simulink model "F16BlockSYM"  (R2012b)
settings: Solver=ode5  StartTime=0.0  StopTime=TFinal  FixedStep=delta_T  RelTol=1e-3
values from neighbouring files (symbols this model uses):
  DisAil_1 = AileronDis    (= 0)    [runF16Sim.m]
  DisAil_2 = -2*AileronDis    (= 0)    [runF16Sim.m]
  DisAil_3 = AileronDis    (= 0)    [runF16Sim.m]
  DisEle_1 = ElevatorDis    (= 0)    [runF16Sim.m]
  DisEle_2 = -2*ElevatorDis    (= 0)    [runF16Sim.m]
  DisEle_3 = ElevatorDis    (= 0)    [runF16Sim.m]
  DisRud_1 = RudderDis    (= 0)    [runF16Sim.m]
  DisRud_2 = -2*RudderDis    (= 0)    [runF16Sim.m]
  DisRud_3 = RudderDis    (= 0)    [runF16Sim.m]
  fi_flag_Simulink = 1    [runF16Sim.m]
  trim_control = [UX(2);UX(5);UX(6)]    [trim_F16_fast.m]
  trim_state = xu(1:13)    [trim_F16_fast.m]
  trim_throttle = UX(1)    [trim_F16_fast.m]
libraries: F16_Actuator_Library x4, aerolibtransform2 x1, aerolibatmos2 x1
settings Model: ExtModeAutoUpdateStatusClock=off  Creator=keviczky  LastModifiedBy=David
settings DataIOCC: Decimation=50  LimitDataPoints=off  SignalLoggingSaveFormat=ModelDataLogs  SignalLoggingName=sigsOut
settings OptimizationCC: BooleanDataType=off  InlineInvariantSignals=on
settings DebuggingCC: SaveWithParameterizedLinksMsg=none  SignalResolutionControl=TryResolveAllWithWarning  SolverPrmCheckMsg=none  MultiTaskDSMMsg=warning  MultiTaskCondExecSysMsg=none  StrictBusMsg=None
settings HardwareCC: TargetUnknown=on
settings RTWCC: IncludeERTFirstTime=on
settings GRTTargetCC: CombineOutputUpdateFcns=off  GRTInterface=on

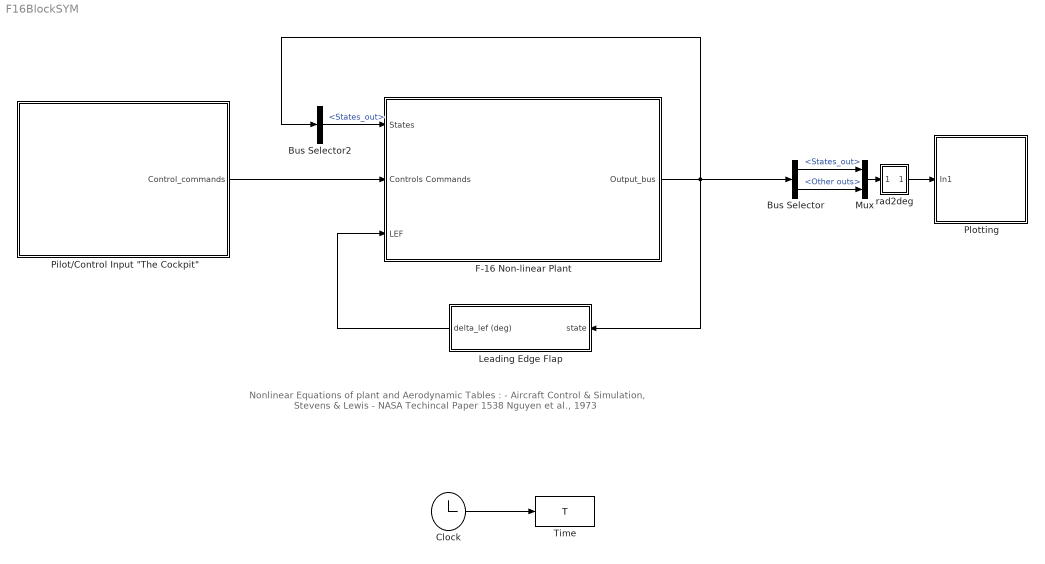
== system F16BlockSYM ==
  note: Nonlinear Equations of plant and Aerodynamic Tables :
      | - Aircraft Control & Simulation, Stevens & Lewis
      | - NASA Techincal Paper 1538 Nguyen et al., 1973
  Bus Selector : BusSelector  OutputSignals=States_out,Other outs
  Bus Selector2 : BusSelector  OutputSignals=States_out
  Clock : Clock
      settings: Decimation=50
  F-16 Non-linear Plant : Subsystem
      mask Display:
      | image(imread('f16.jpg'))
      | port_label('output', 1, 'Out_bus')
      | port_label('input', 1, 'State_feedback')
      | port_label('input', 2, 'Control_Commands')
      | port_label('input', 3, 'LEF_def')
  Leading Edge Flap : Subsystem
  Mux : Mux  Inputs=2
  "Pilot/Control Input \"The Cockpit\"" : Subsystem
      mask Display:
      | image(imread('F-16-Cockpit.jpg'))
      | port_label('output', 1, 'Control_commands')
  Plotting : Subsystem
      mask Display: image(imread('f16output.jpg'))
  Time : ToWorkspace  VariableName=T  SampleTime=-1
      settings: Decimation=100
  rad2deg : Subsystem
  wires:
  "Pilot/Control Input \"The Cockpit\""/1(Control_commands) -> F-16 Non-linear Plant/2(Controls Commands)
  Clock/1 -> Time/1
  rad2deg/1(Out1) -> Plotting/1(In1)
  Bus Selector/1 -> Mux/1  "<States_out>"
  Bus Selector/2 -> Mux/2  "<Other outs>"
  Mux/1 -> rad2deg/1(In1)
  F-16 Non-linear Plant/1(Output_bus) -> Leading Edge Flap/1(state), Bus Selector2/1, Bus Selector/1
  Bus Selector2/1 -> F-16 Non-linear Plant/1(States)  "<States_out>"
  Leading Edge Flap/1(delta_lef (deg)) -> F-16 Non-linear Plant/3(LEF)

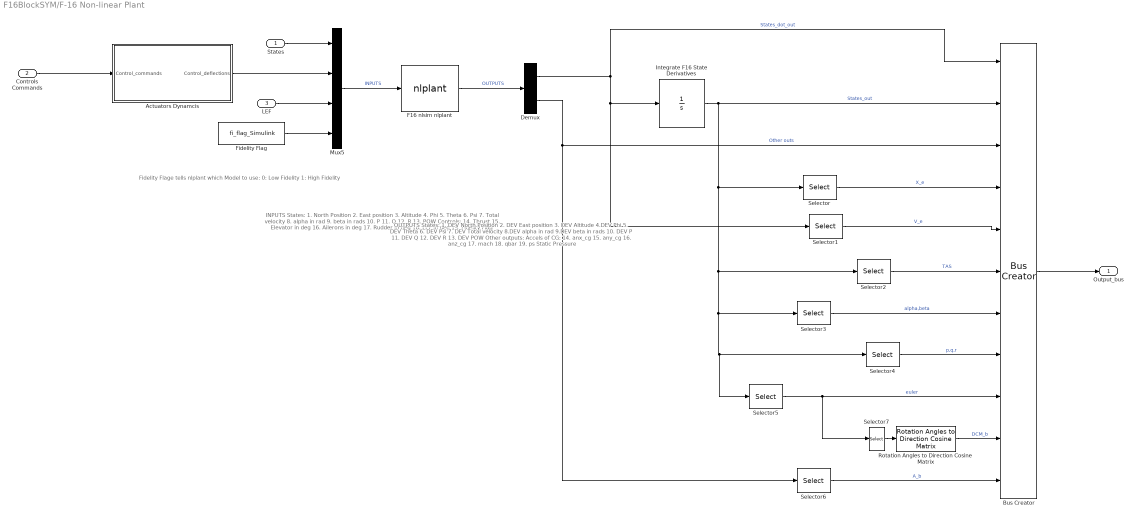
== system F16BlockSYM/F-16 Non-linear Plant ==
  note: INPUTS
      | States:
      | 1. North Position
      | 2. East position
      | 3. Altitude
      | 4. Phi
      | 5. Theta
      | 6. Psi
      | 7. Total velocity
      | 8. alpha in rad
      | 9. beta in rads
      | 10. P
      | 11. Q
      | 12. R
      | 13. POW
      |
      | Controls:
      | 14. Thrust
      | 15. Elevator in deg
      | 16. Ailerons in deg
      | 17. Rudder in deg
      | 18. LEF in deg
      |
      | 19. Fidelity Flag
  note: OUTPUTS
      | States:
      | 1. DEV North Position
      | 2. DEV East position
      | 3. DEV Altitude
      | 4.DEV  Phi
      | 5. DEV Theta
      | 6. DEV Psi
      | 7. DEV Total velocity
      | 8.DEV alpha in rad
      | 9.DEV  beta in rads
      | 10. DEV P
      | 11. DEV Q
      | 12. DEV R
      | 13. DEV POW
      |
      | Other outputs:
      | Accels of CG:
      | 14. anx_cg
      | 15. any_cg
      | 16. anz_cg
      | 17. mach
      | 18. qbar
      | 19. ps   Static Pressure
  note: Fidelity Flage tells nlplant
      | which Model to use:
      | 0: Low Fidelity
      | 1: High Fidelity
  States : Inport
  Controls Commands : Inport  Port=2
  LEF : Inport  Port=3
  Actuators Dynamcis : Subsystem  TreatAsAtomicUnit=on
  Bus Creator : BusCreator  Inputs=11
  Demux : Demux  Outputs=[13 6]
  F16 nlsim nlplant : MATLABFcn  MATLABFcn=nlplant  OutputDimensions=19  OutputSignalType=real
  Fidelity Flag : Constant  Value=fi_flag_Simulink
  Integrate F16 State Derivatives : Integrator  InitialCondition=trim_state
  Mux5 : Mux  Inputs=[13 4 1 1]
  Rotation Angles to Direction Cosine Matrix : aerolibtransform2/Rotation Angles to Direction Cosine Matrix  rotationOrder=ZYX
  Selector : Selector  InputPortWidth=13  IndexOptions=Index vector (dialog)  Indices=[1:3]  OutputSizes=1
  Selector1 : Selector  InputPortWidth=13  IndexOptions=Index vector (dialog)  Indices=[1:3]  OutputSizes=1
  Selector2 : Selector  InputPortWidth=13  IndexOptions=Index vector (dialog)  Indices=[7]  OutputSizes=1
  Selector3 : Selector  InputPortWidth=13  IndexOptions=Index vector (dialog)  Indices=[8:9]  OutputSizes=1
  Selector4 : Selector  InputPortWidth=13  IndexOptions=Index vector (dialog)  Indices=[10:12]  OutputSizes=1
  Selector5 : Selector  InputPortWidth=13  IndexOptions=Index vector (dialog)  Indices=[4:6]  OutputSizes=1
  Selector6 : Selector  InputPortWidth=6  IndexOptions=Index vector (dialog)  Indices=[1:3]  OutputSizes=1
  Selector7 : Selector  InputPortWidth=3  IndexOptions=Index vector (dialog)  Indices=[3 2 1]  OutputSizes=1
  Output_bus : Outport
  wires:
  Demux/1 -> Selector1/1, Integrate F16 State Derivatives/1, Bus Creator/1  "States_dot_out"
  Selector/1 -> Bus Creator/4  "X_e"
  Selector1/1 -> Bus Creator/5  "V_e"
  Selector2/1 -> Bus Creator/6  "TAS"
  Selector3/1 -> Bus Creator/7  "alpha,beta"
  Selector4/1 -> Bus Creator/8  "p,q,r"
  Selector5/1 -> Selector7/1, Bus Creator/9  "euler"
  Selector6/1 -> Bus Creator/11  "A_b"
  Demux/2 -> Selector6/1, Bus Creator/3  "Other outs"
  Selector7/1 -> Rotation Angles to Direction Cosine Matrix/1
  Integrate F16 State Derivatives/1 -> Selector5/1, Selector4/1, Selector3/1, Selector2/1, Selector/1, Bus Creator/2  "States_out"
  Rotation Angles to Direction Cosine Matrix/1 -> Bus Creator/10  "DCM_b"
  Bus Creator/1 -> Output_bus/1
  Fidelity Flag/1 -> Mux5/4
  LEF/1 -> Mux5/3
  Controls Commands/1 -> Actuators Dynamcis/1(Control_commands)
  States/1 -> Mux5/1
  Mux5/1 -> F16 nlsim nlplant/1  "INPUTS"
  F16 nlsim nlplant/1 -> Demux/1  "OUTPUTS"
  Actuators Dynamcis/1(Control_deflections) -> Mux5/2

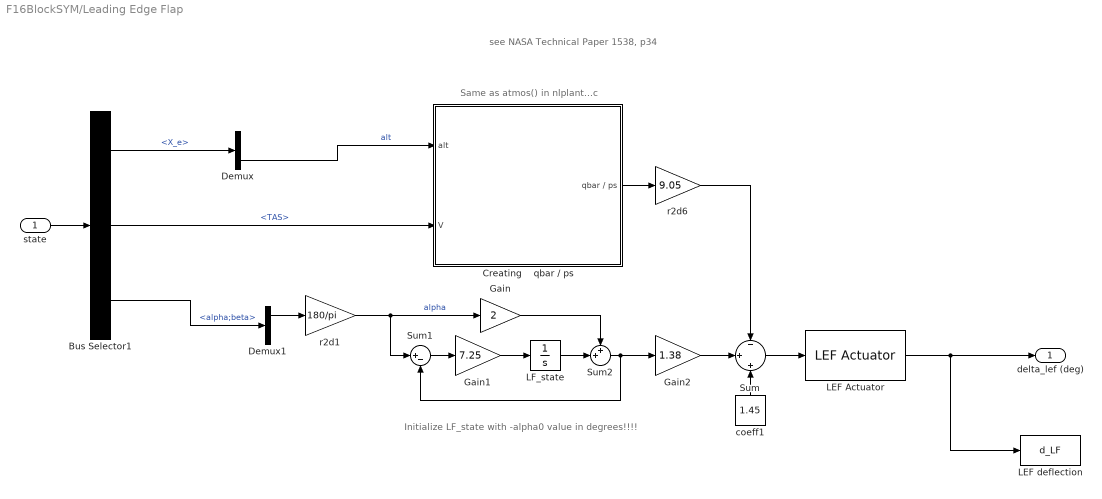
== system F16BlockSYM/Leading Edge Flap ==
  note: see NASA Technical Paper 1538, p34
  note: Same as atmos() in nlplant...c
  note: Initialize LF_state with -alpha0 value in degrees!!!!
  state : Inport
  Bus Selector1 : BusSelector  OutputSignals=X_e,TAS,alpha;beta
  Creating    qbar / ps : Subsystem
  Demux : Demux  Outputs=3
  Demux1 : Demux  Outputs=2
  Gain : Gain  Gain=2  SaturateOnIntegerOverflow=on  OutDataTypeStr=Inherit: Same as input  ParamDataTypeStr=Inherit: Same as input
  Gain1 : Gain  Gain=7.25  SaturateOnIntegerOverflow=on  OutDataTypeStr=Inherit: Same as input  ParamDataTypeStr=Inherit: Same as input
  Gain2 : Gain  Gain=1.38  SaturateOnIntegerOverflow=on  OutDataTypeStr=Inherit: Same as input  ParamDataTypeStr=Inherit: Same as input
  LEF Actuator : F16_Actuator_Library/LEF Actuator
  LEF deflection : ToWorkspace  VariableName=d_LF  SampleTime=-1
      settings: Decimation=100
  LF_state : Integrator  InitialCondition=-trim_state(8)*180/pi
  Sum : Sum  Inputs=-|+|+  SaturateOnIntegerOverflow=on  InputSameDT=on  OutDataTypeStr=Inherit: Same as first input
  Sum1 : Sum  Inputs=|+-  SaturateOnIntegerOverflow=on  InputSameDT=on  OutDataTypeStr=Inherit: Same as first input
  Sum2 : Sum  Inputs=++|  SaturateOnIntegerOverflow=on  InputSameDT=on  OutDataTypeStr=Inherit: Same as first input
  coeff1 : Constant  Value=1.45
  r2d1 : Gain  Gain=180/pi  SaturateOnIntegerOverflow=on  OutDataTypeStr=Inherit: Same as input  ParamDataTypeStr=Inherit: Same as input
  r2d6 : Gain  Gain=9.05  SaturateOnIntegerOverflow=on  OutDataTypeStr=Inherit: Same as input  ParamDataTypeStr=Inherit: Same as input
  delta_lef (deg) : Outport
  wires:
  LEF Actuator/1 -> LEF deflection/1, delta_lef (deg)/1
  Sum/1 -> LEF Actuator/1
  state/1 -> Bus Selector1/1
  Sum1/1 -> Gain1/1
  Gain1/1 -> LF_state/1
  Gain/1 -> Sum2/1
  Gain2/1 -> Sum/2
  Demux1/1 -> r2d1/1
  coeff1/1 -> Sum/3
  Sum2/1 -> Sum1/2, Gain2/1
  LF_state/1 -> Sum2/2
  r2d1/1 -> Sum1/1, Gain/1  "alpha"
  Bus Selector1/2 -> Creating    qbar / ps/2(V)  "<TAS>"
  Creating    qbar / ps/1(qbar / ps) -> r2d6/1
  r2d6/1 -> Sum/1
  Demux/3 -> Creating    qbar / ps/1(alt)  "alt"
  Bus Selector1/1 -> Demux/1  "<X_e>"
  Bus Selector1/3 -> Demux1/1  "<alpha;beta>"

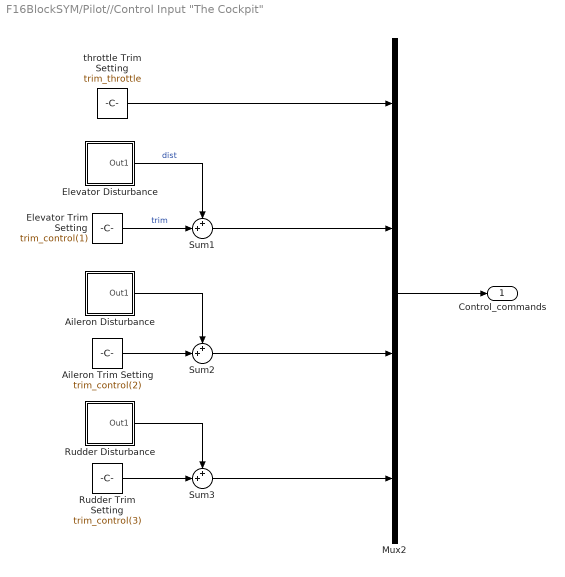
== system F16BlockSYM/Pilot//Control Input "The Cockpit" ==
  Aileron Disturbance : Subsystem
  Aileron Trim Setting : Constant  Value=trim_control(2)
  Elevator Disturbance : Subsystem
  Elevator Trim Setting : Constant  Value=trim_control(1)  VectorParams1D=off
  Mux2 : Mux
  Rudder Disturbance : Subsystem
  Rudder Trim Setting : Constant  Value=trim_control(3)
  Sum1 : Sum  Inputs=++|  SaturateOnIntegerOverflow=on  InputSameDT=on  OutDataTypeStr=Inherit: Same as first input
  Sum2 : Sum  Inputs=++|  SaturateOnIntegerOverflow=on  InputSameDT=on  OutDataTypeStr=Inherit: Same as first input
  Sum3 : Sum  Inputs=++|  SaturateOnIntegerOverflow=on  InputSameDT=on  OutDataTypeStr=Inherit: Same as first input
  throttle Trim Setting : Constant  Value=trim_throttle
  Control_commands : Outport
  wires:
  throttle Trim Setting/1 -> Mux2/1
  Elevator Trim Setting/1 -> Sum1/2  "trim"
  Sum2/1 -> Mux2/3
  Aileron Trim Setting/1 -> Sum2/2
  Sum3/1 -> Mux2/4
  Rudder Trim Setting/1 -> Sum3/2
  Mux2/1 -> Control_commands/1
  Elevator Disturbance/1(Out1) -> Sum1/1  "dist"
  Aileron Disturbance/1(Out1) -> Sum2/1
  Rudder Disturbance/1(Out1) -> Sum3/1
  Sum1/1 -> Mux2/2

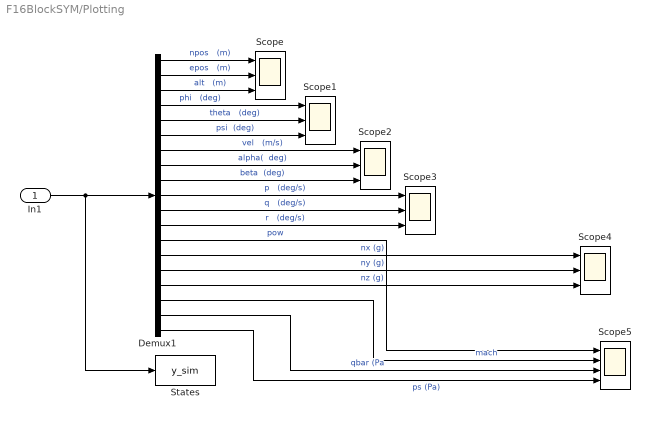
== system F16BlockSYM/Plotting ==
  In1 : Inport
  Demux1 : Demux  Outputs=19
  Scope{,1..4} (5 alike) : Scope  NumInputPorts=3
      Scope settings: YMin=12100~6e-11~13235  YMax=13700~8.75e-11~13320  Decimation=20
      Scope1 settings: TimeRange=10  YMin=-0.000525~3.88949~-0.00034  YMax=-0.000465~3.88952~-0.000275  Decimation=20
      Scope2 settings: YMin=160~3.89041~-0.337005  YMax=160.001~3.89042~-0.337004  SaveName=ScopeData2  Decimation=20
      Scope3 settings: YMin=-5~-5~-5  YMax=5~5~5  SaveName=ScopeData3  Decimation=20
      Scope4 settings: YMin=-5~-5~-5  YMax=5~5~5  SaveName=ScopeData4  Decimation=20
  Scope5 : Scope  NumInputPorts=4
      settings: ShowLegends=on  YMin=13.2562~0.495~10000~58450  YMax=13.2562~0.507~10600~58900  SaveName=ScopeData5
  States : ToWorkspace  VariableName=y_sim  SampleTime=-1
      settings: Decimation=100
  wires:
  Demux1/1 -> Scope/1  "npos   (m)"
  Demux1/2 -> Scope/2  "epos   (m)"
  Demux1/3 -> Scope/3  "alt   (m)"
  Demux1/5 -> Scope1/2  "theta   (deg)"
  Demux1/6 -> Scope1/3  "psi  (deg)"
  Demux1/7 -> Scope2/1  "vel   (m/s)"
  Demux1/8 -> Scope2/2  "alpha(  deg)"
  Demux1/9 -> Scope2/3  "beta  (deg)"
  Demux1/10 -> Scope3/1  "p   (deg/s)"
  Demux1/11 -> Scope3/2  "q   (deg/s)"
  Demux1/12 -> Scope3/3  "r   (deg/s)"
  Demux1/14 -> Scope4/1  "nx (g)"
  Demux1/15 -> Scope4/2  "ny (g)"
  Demux1/16 -> Scope4/3  "nz (g)"
  Demux1/4 -> Scope1/1  "phi   (deg)"
  Demux1/17 -> Scope5/2  "mach"
  Demux1/18 -> Scope5/3  "qbar (Pa"
  Demux1/19 -> Scope5/4  "ps (Pa)"
  In1/1 -> Demux1/1, States/1
  Demux1/13 -> Scope5/1  "pow"

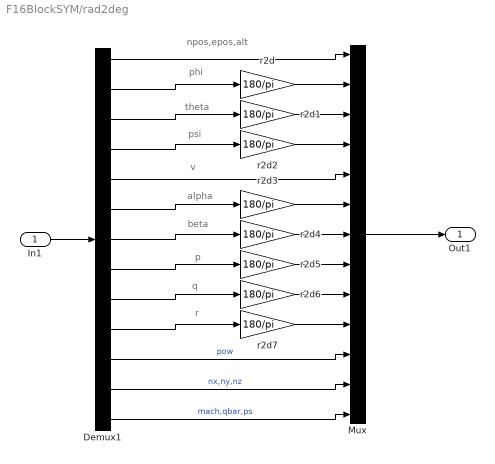
== system F16BlockSYM/rad2deg ==
  note: npos,epos,alt
  note: phi
  note: theta
  note: psi
  note: v
  note: alpha
  note: beta
  note: p
  note: q
  note: r
  In1 : Inport
  Demux1 : Demux  Outputs=[3 1 1 1 1 1 1 1 1 1 1 3 3]
  Mux : Mux  Inputs=[3 1 1 1 1 1 1 1 1 1 1 3 3]
  r2d{,1..7} (8 alike) : Gain  Gain=180/pi  SaturateOnIntegerOverflow=on  OutDataTypeStr=Inherit: Same as input  ParamDataTypeStr=Inherit: Same as input
  Out1 : Outport
  wires:
  In1/1 -> Demux1/1
  Demux1/2 -> r2d/1
  Demux1/3 -> r2d1/1
  Demux1/4 -> r2d2/1
  Demux1/1 -> Mux/1
  Demux1/5 -> Mux/5
  r2d2/1 -> Mux/4
  r2d1/1 -> Mux/3
  r2d/1 -> Mux/2
  Demux1/6 -> r2d3/1
  Demux1/7 -> r2d4/1
  Demux1/8 -> r2d5/1
  Demux1/9 -> r2d6/1
  Demux1/10 -> r2d7/1
  r2d4/1 -> Mux/7
  r2d5/1 -> Mux/8
  r2d6/1 -> Mux/9
  r2d7/1 -> Mux/10
  Mux/1 -> Out1/1
  Demux1/12 -> Mux/12  "nx,ny,nz"
  Demux1/13 -> Mux/13  "mach,qbar,ps"
  r2d3/1 -> Mux/6
  Demux1/11 -> Mux/11  "pow"

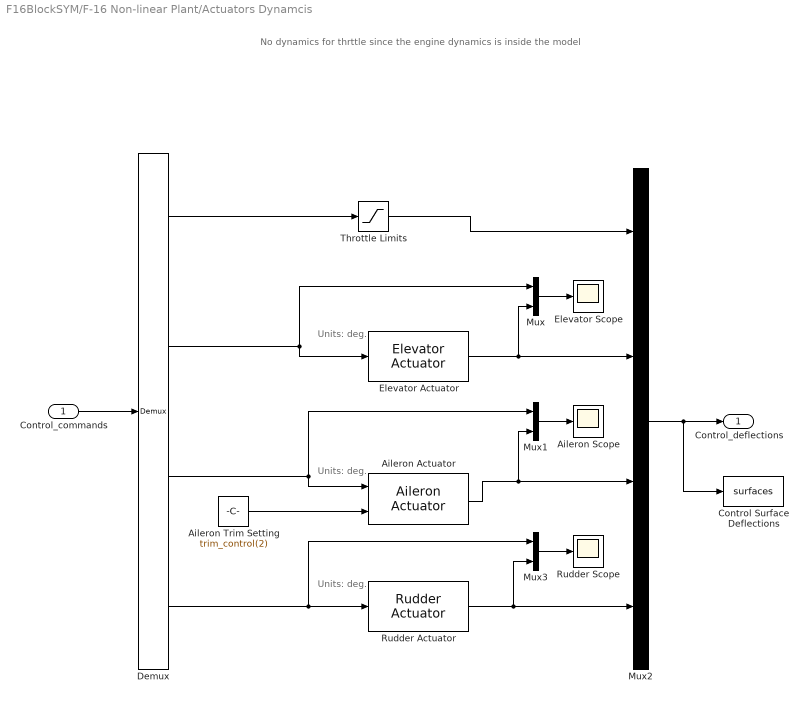
== system F16BlockSYM/F-16 Non-linear Plant/Actuators Dynamcis ==
  note: No dynamics for thrttle since the engine dynamics is inside the model
  note: Units: deg.
  note: Units: deg.
  note: Units: deg.
  Control_commands : Inport
  Aileron Actuator : F16_Actuator_Library/Aileron Actuator
  Aileron Scope : Scope
      settings: TimeRange=30  SaveName=ScopeData9
  Aileron Trim Setting : Constant  Value=trim_control(2)
  Control Surface Deflections : ToWorkspace  VariableName=surfaces  SampleTime=-1
      settings: Decimation=100
  Demux : Demux
  Elevator Actuator : F16_Actuator_Library/Elevator Actuator
  Elevator Scope : Scope
      settings: TimeRange=5  YMin=-2.05537  YMax=-2.05537  SaveName=ScopeData10
  Mux : Mux  Inputs=2
  Mux1 : Mux  Inputs=2
  Mux2 : Mux
  Mux3 : Mux  Inputs=2
  Rudder Actuator : F16_Actuator_Library/Rudder Actuator
  Rudder Scope : Scope
      settings: YMin=0.0727808  YMax=0.0727808  SaveName=ScopeData11
  Throttle Limits : Saturate  UpperLimit=1  LowerLimit=0
  Control_deflections : Outport
  wires:
  Demux/2 -> Elevator Actuator/1, Mux/1
  Demux/3 -> Aileron Actuator/1, Mux1/1
  Demux/4 -> Mux3/1, Rudder Actuator/1
  Mux2/1 -> Control_deflections/1, Control Surface Deflections/1
  Elevator Actuator/1 -> Mux2/2, Mux/2
  Aileron Actuator/1 -> Mux2/3, Mux1/2
  Rudder Actuator/1 -> Mux2/4, Mux3/2
  Mux1/1 -> Aileron Scope/1
  Mux3/1 -> Rudder Scope/1
  Control_commands/1 -> Demux/1
  Demux/1 -> Throttle Limits/1
  Mux/1 -> Elevator Scope/1
  Throttle Limits/1 -> Mux2/1
  Aileron Trim Setting/1 -> Aileron Actuator/2

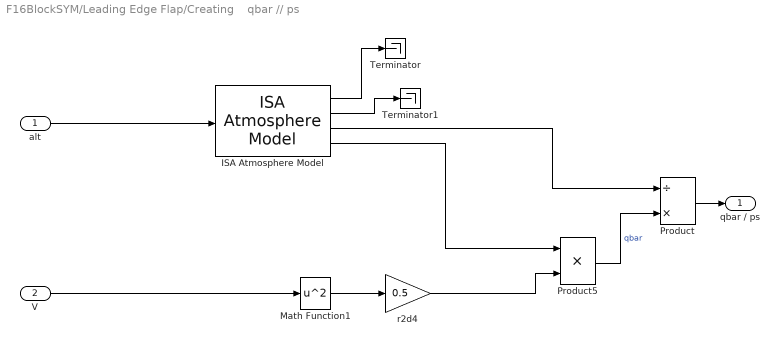
== system F16BlockSYM/Leading Edge Flap/Creating    qbar // ps ==
  alt : Inport
  V : Inport  Port=2
  ISA Atmosphere Model : aerolibatmos2/ISA Atmosphere Model  custom=off  g=9.80665  gamma=1.4  R=287.0531  L=0.0065  h_trop=11000  h_strat=20000  rho0=1.225  P0=101325  T0=288.15
  Math Function1 : Math  Operator=square  SaturateOnIntegerOverflow=on
  Product : Product  Inputs=/*  SaturateOnIntegerOverflow=on  InputSameDT=on  OutDataTypeStr=Inherit: Same as first input
  Product5 : Product  Inputs=**  SaturateOnIntegerOverflow=on  InputSameDT=on  OutDataTypeStr=Inherit: Same as first input
  Terminator : Terminator
  Terminator1 : Terminator
  r2d4 : Gain  Gain=0.5  SaturateOnIntegerOverflow=on  OutDataTypeStr=Inherit: Same as input  ParamDataTypeStr=Inherit: Same as input
  qbar / ps : Outport
  wires:
  alt/1 -> ISA Atmosphere Model/1
  Math Function1/1 -> r2d4/1
  r2d4/1 -> Product5/2
  Product5/1 -> Product/2  "qbar"
  V/1 -> Math Function1/1
  Product/1 -> qbar / ps/1
  ISA Atmosphere Model/4 -> Product5/1
  ISA Atmosphere Model/3 -> Product/1
  ISA Atmosphere Model/1 -> Terminator/1
  ISA Atmosphere Model/2 -> Terminator1/1

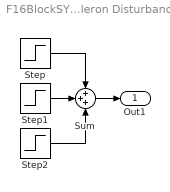
== system F16BlockSYM/Pilot//Control Input "The Cockpit"/Aileron Disturbance ==
  Step : Step  After=DisAil_1  SampleTime=0
  Step1 : Step  Time=3  After=DisAil_2  SampleTime=0
  Step2 : Step  Time=5  After=DisAil_3  SampleTime=0
  Sum : Sum  Inputs=+++  SaturateOnIntegerOverflow=on  InputSameDT=on  OutDataTypeStr=Inherit: Same as first input
  Out1 : Outport
  wires:
  Step1/1 -> Sum/2
  Step/1 -> Sum/1
  Step2/1 -> Sum/3
  Sum/1 -> Out1/1

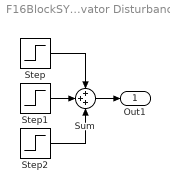
== system F16BlockSYM/Pilot//Control Input "The Cockpit"/Elevator Disturbance ==
  Step : Step  After=DisEle_1  SampleTime=0
  Step1 : Step  Time=3  After=DisEle_2  SampleTime=0
  Step2 : Step  Time=5  After=DisEle_3  SampleTime=0
  Sum : Sum  Inputs=+++  SaturateOnIntegerOverflow=on  InputSameDT=on  OutDataTypeStr=Inherit: Same as first input
  Out1 : Outport
  wires:
  Step1/1 -> Sum/2
  Step/1 -> Sum/1
  Step2/1 -> Sum/3
  Sum/1 -> Out1/1

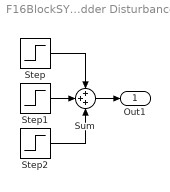
== system F16BlockSYM/Pilot//Control Input "The Cockpit"/Rudder Disturbance ==
  Step : Step  After=DisRud_1  SampleTime=0
  Step1 : Step  Time=3  After=DisRud_2  SampleTime=0
  Step2 : Step  Time=5  After=DisRud_3  SampleTime=0
  Sum : Sum  Inputs=+++  SaturateOnIntegerOverflow=on  InputSameDT=on  OutDataTypeStr=Inherit: Same as first input
  Out1 : Outport
  wires:
  Step1/1 -> Sum/2
  Step/1 -> Sum/1
  Step2/1 -> Sum/3
  Sum/1 -> Out1/1
